simulink model "nc_pendulum"  (R2018a)
settings: Solver=VariableStepAuto  StartTime=0.0  StopTime=inf  FixedStep=r  RelTol=1e-3
libraries: aerolibanimutils x1
settings Model: Creator=ncrosty  LastModifiedBy=ncrosty
settings SolverCC: AlgebraicLoopSolver=LineSearch
settings RTWCC: TargetLang=C++
settings GRTTargetCC: TargetLangStandard=C++03 (ISO)  MultiInstanceERTCode=on  CodeInterfacePackaging=C++ class

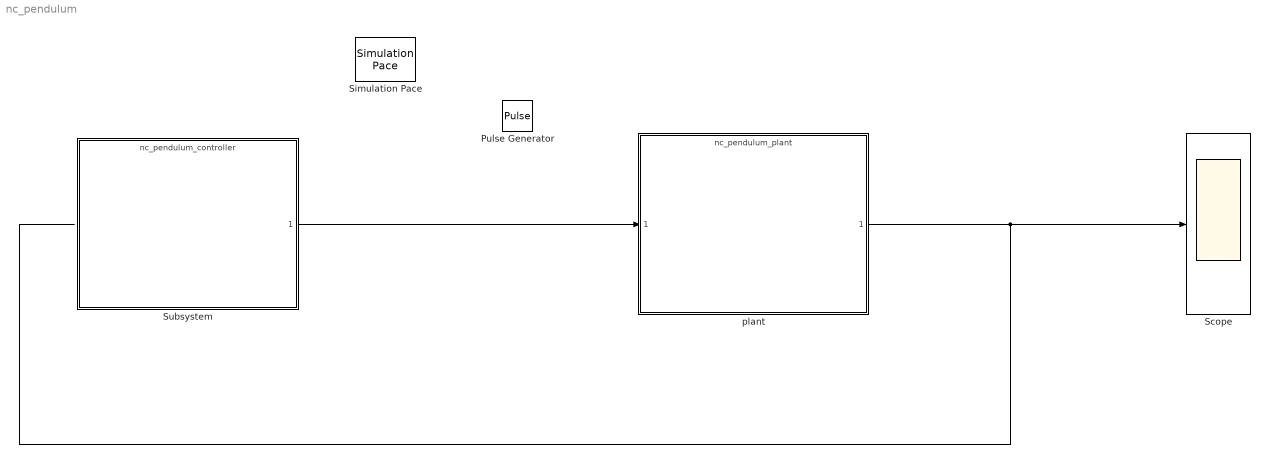
== system nc_pendulum ==
  Pulse Generator : DiscretePulseGenerator  PulseType=Time based  Period=10  PulseWidth=5
  Scope : Scope
  Simulation Pace : aerolibanimutils/Simulation Pace  SimulationPace=1  SleepMode=MATLAB Thread  OutputPaceError=off  SampleTime=1/30
  Subsystem : ModelReference  ModelNameDialog=nc_pendulum_controller  SimulationMode=Normal  ModelReferenceVersion=1.204
  plant : ModelReference  ModelNameDialog=nc_pendulum_plant  SimulationMode=Normal  ModelReferenceVersion=1.46
  wires:
  plant/1 -> Scope/1
  Subsystem/1 -> plant/1
